simulink model "rtlsdr_fm_fdm_demod"  (R2014b)
settings: Solver=ode45  StartTime=0.0  StopTime=60  RelTol=1e-3
PreLoadFcn:
  | %%%%%%%%%%%%%%%%%%%%%%%%%%%%%%%%%%%%%%%%%%%%%%%%%%%%%%%%%%%%%%%%%%%%%%%%%%%
  | % check to see if Simulink library folder is missing from the MATLAB path %
  | %%%%%%%%%%%%%%%%%%%%%%%%%%%%%%%%%%%%%%%%%%%%%%%%%%%%%%%%%%%%%%%%%%%%%%%%%%%
  | if isempty(strfind(path, 'rtlsdr_book_library'))
  | 
  |     % create error window
  |     fig_error = figure(...
  |         'Name', 'Error: RTL-SDR Book Library',...
  |         'Toolbar','none',...
  |         'MenuBar','none',...
  |         'NumberTitle','off',...
  |         'Resize','off',...
  |         'WindowStyle','modal');
  |     fig_error.Position(3) = 600;
  |     fig_error.Position(4) = 150;
  |     fig_axes = axes(...
  |         'Parent',fig_error,...
  |         'Position',[0,0,1,1],...
  |         'visible','off');
  |     % error message
  |     t_title = text(.05,.8,...
  |         'MISSING DIRECTORIES',...
  |         'FontSize',11.5);
  |     t_body = text(.075,.6,...
  |         [{'Simulink cannot find the  \it{<root>}\rm / \it{rtlsdr\_book\_library}\rm  folder in the \it{MATLAB Path}\rm.'},...
  |         {'Please set the MATLAB path following the instructions given in Exercise 2.4.'}],...
  |         'FontSize',10.5);
  |     % buttons
  |     btn_path = uicontrol(...
  |         'Parent',fig_error,...
  |         'String','Set Path Now',...
  |         'FontSize',10,...
  |         'Callback', 'pathtool; close(fig_error);',...
  |         'Position', [fig_error.Position(3)/2-210, 30, 200, 30]);
  |     btn_abort = uicontrol(...
  |         'Parent',fig_error,...
  |         'String','No thanks',...
  |         'FontSize',10,...
  |         'Callback', 'close(fig_error); abort=1;',...
  |         'Position', [fig_error.Position(3)/2+10, 30, 200, 30]);
  | 
  |     % pause to allow user to interact with error box
  |     uiwait(fig_error);
  | 
  |     % abort simulation
  |     try
  |         if abort==1
  |             set_param(gcs, 'SimulationCommand', 'stop');
  |         end
  |     end
  | 
  |     % if user has set path, allow diagram to be updated
  |     if ~exist('abort','var')
  |         % create error window
  |         fig_update = figure(...
  |             'Name', 'Update Diagram',...
  |             'Toolbar','none',...
  |             'MenuBar','none',...
  |             'NumberTitle','off',...
  |             'Resize','off');
  |         fig_update.Position(3) = 400;
  |         fig_update.Position(4) = 120;
  |         fig_axes = axes(...
  |             'Parent',fig_update,...
  |             'Position',[0,0,1,1],...
  |             'visible','off');
  |         % instruction message
  |         t_body = text(.075,.7,...
  |             'Once you have set the path, update the block diagram',...
  |             'FontSize',10.5);
  |         % button
  |         btn_update = uicontrol(...
  |             'Parent',fig_update,...
  |             'String','Update Block Diagram',...
  |             'FontSize',10,...
  |             'Callback', 'set_param(gcs,''SimulationCommand'',''update''); close(gcf)',...
  |             'Position', [fig_update.Position(3)/2-100, 30, 200, 30]);
  |     end
  | 
  |     % clear error components
  |     clear('fig_error','fig_update','fig_axes','t_title','t_body','btn_path','btn_abort','btn_update','abort');
  | 
  | end
  | %%%%%%%%%%%%%%%%%%%%%%%%%%%%%%%%%%%%%%%%%%%%%%%%%%%%%%%%%%%%%%%%%%%%%%%%%%%
undefined symbols (not defined in the file or in its folder): dfilt, fdesignblkfcn, gcbh, startfcn_spectrum_analyzer
libraries: dsparch4 x5, rtlsdr_book_library x4, dspmlti4 x3, sdrrlib x1, dspsnks4 x1
CloseFcn:
  | closefcn_model
Description:
  | Software, Simulation Examples and Design Exercises Licence Agreement
  | 
  | This license agreement refers to the simulation examples, design exercises and files,
  | and associated software MATLAB and Simulink resources that accompany the book:
  | 
  |      Title: Software Defined Radio using MATLAB & Simulink and the RTL-SDR
  |      Published by Strathclyde Academic Media, 2015
  |      Authored by Robert W. Stewart, Kenneth W. Barlee, Dale S.W. Atkinson,
  |      and Louise H. Crockett
  | 
  | and made available as a download from, www.desktopSDR.com or variously acquired
  | by other means such as via USB storage, cloud storage, disk or any other electronic
  | or optical or magnetic storage mechanism. These files and associated software may
  | be used subject to the terms of agreement of the conditions below:
  | 
  |     Copyright © 2015 Robert W. Stewart, Kenneth W. Barlee, Dale S.W. Atkinson,
  |     and Louise H. Crockett
  |     All rights reserved.
  | 
  | Redistribution and use in source and binary forms, with or without modification, are
  | permitted provided that the following conditions are met:
  | 
  |    1.  Redistributions of source code must retain the above copyright notice, this list of
  |         conditions and the following disclaimer.
  | 
  |    2.  Redistributions in binary form must reproduce the above copyright notice, this
  |         list of conditions and the following disclaimer in the documentation and/or other
  |         materials provided with the distribution.
  | 
  |    3.  Neither the name of the copyright holder nor the names of its contributors may
  |         be used to endorse or promote products derived from this software without
  |         specific prior written permission.
  | 
  |    4.  In all cases, the software is, and all modifications and derivatives of the
  |         software shall be, licensed to you solely for use in conjunction with The
  |         MathWorks, Inc. products and service offerings.
  | 
  | THIS SOFTWARE IS PROVIDED BY THE COPYRIGHT HOLDERS AND CONTRIBUTORS
  | "AS IS" AND ANY EXPRESS OR IMPLIED WARRANTIES, INCLUDING, BUT NOT LIMITED
  | TO, THE IMPLIED WARRANTIES OF MERCHANTABILITY AND FITNESS FOR A
  | PARTICULAR PURPOSE ARE DISCLAIMED. IN NO EVENT SHALL THE COPYRIGHT
  | HOLDER OR CONTRIBUTORS BE LIABLE FOR ANY DIRECT, INDIRECT, INCIDENTAL,
  | SPECIAL, EXEMPLARY, OR CONSEQUENTIAL DAMAGES (INCLUDING, BUT NOT
  | LIMITED TO, PROCUREMENT OF SUBSTITUTE GOODS OR SERVICES; LOSS OF USE,
  | DATA, OR PROFITS; OR BUSINESS INTERRUPTION) HOWEVER CAUSED AND ON ANY
  | THEORY OF LIABILITY, WHETHER IN CONTRACT, STRICT LIABILITY, OR TORT
  | (INCLUDING NEGLIGENCE OR OTHERWISE) ARISING IN ANY WAY OUT OF THE USE
  | OF THIS SOFTWARE, EVEN IF ADVISED OF THE POSSIBILITY OF SUCH DAMAGE.
  | 
  | 
  | Audio Tracks used in Simulations Examples and Design Exercises
  | 
  | The music and vocal files used within the Examples files and software within the book
  | were variously written, arranged, performed, recorded and produced by Garrey Rice,
  | Adam Struth, Jamie Struth, Iain Thistlethwaite and also Marshall Craigmyle who
  | collectively, and individually where appropriate, assert and retain all of their copyright,
  | performance and artistic rights. Permission to use and reproduce this music is
  | granted for all purposes associated with MATLAB and Simulink software and the
  | simulation examples and design exercises files that accompany this book. Requests to
  | use the music for any other purpose should be directed to: info@desktopSDR.com.
  | For information on music track names, full credits, and links to the musicians please
  | refer to www.desktopSDR.com/more/audio.
settings Model: SimulationMode=accelerator  Creator=desktopSDR Team  LastModifiedBy=desktopSDR Team
settings DataIOCC: LimitDataPoints=off  SaveOutput=off  SignalLogging=off  SaveTime=off

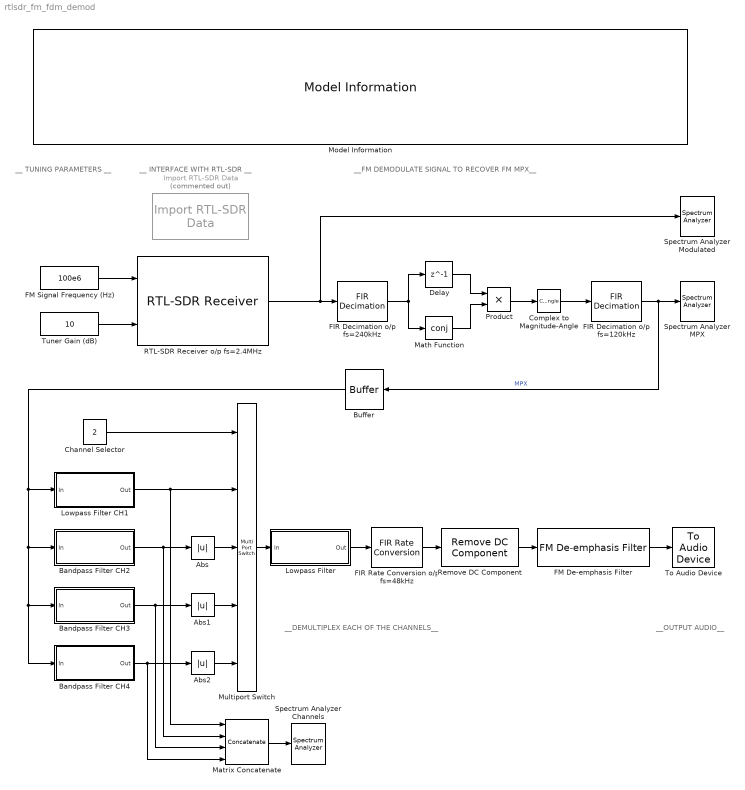
== system rtlsdr_fm_fdm_demod ==
  note: __ TUNING PARAMETERS __
  note: __ INTERFACE WITH RTL-SDR __
  note: __OUTPUT AUDIO__
  note: __FM DEMODULATE SIGNAL TO RECOVER FM MPX__
  note: __DEMULTIPLEX EACH OF THE CHANNELS__
  Abs : Abs
  Abs1 : Abs
  Abs2 : Abs
  Bandpass Filter CH2 : Subsystem  DialogController=fdesignblkfcn  InitFcn=fdesignblkfcn(gcbh, {'InitFcn'});  mask(Bandpass Filter){}
      mask help: Design a bandpass filter
      settings: CopyFcn=fdesignblkfcn(gcbh, {'CopyFcn'});
      mask Help: helpview(mapfilelocation('dsp'), 'dspbandpassfilter');
      mask Display: disp('Bandpass');
  Bandpass Filter CH3 : Subsystem  DialogController=fdesignblkfcn  InitFcn=fdesignblkfcn(gcbh, {'InitFcn'});  mask(Bandpass Filter){}
      mask help: Design a bandpass filter
      settings: CopyFcn=fdesignblkfcn(gcbh, {'CopyFcn'});
      mask Help: helpview(mapfilelocation('dsp'), 'dspbandpassfilter');
      mask Display: disp('Bandpass');
  Bandpass Filter CH4 : Subsystem  DialogController=fdesignblkfcn  InitFcn=fdesignblkfcn(gcbh, {'InitFcn'});  mask(Bandpass Filter){}
      mask help: Design a bandpass filter
      settings: CopyFcn=fdesignblkfcn(gcbh, {'CopyFcn'});
      mask Help: helpview(mapfilelocation('dsp'), 'dspbandpassfilter');
      mask Display: disp('Bandpass');
  Buffer : Buffer  N=4000  TreatMby1Signals=One channel
  Channel Selector : Constant  Value=2
  Complex to Magnitude-Angle : ComplexToMagnitudeAngle  Output=Angle
  Delay : Delay  DelayLength=1  InitialCondition=0  InputProcessing=Columns as channels (frame based)
  FIR Decimation o/p fs=120kHz : dspmlti4/FIR Decimation  h=firpm(150, [0 53e3 60e3 (240e3/2)]/(240e3/2), [1 1 0 0], [1 1],20)  D=2  filtStruct=Direct form  framing=Allow multirate processing  inputOffset=0  outputBufInitCond=0  InputProcessing=Columns as channels (frame based)  firstCoeffDataTypeStr=Inherit: Same word length as input  firstCoeffLastDataTypeStr=Inherit: Same word length as input  firstCoeffMin=[]  firstCoeffMax=[]  outputDataTypeStr=Inherit: Same as accumulator  outputLastDataTypeStr=Inherit: Same as accumulator  outputMin=[]  outputMax=[]  roundingMode=Floor  overflowMode=off  FilterSource=Specify via dialog  FilterObject=Hm_firdecim
      settings: allowOverrides=off
  FIR Decimation o/p fs=240kHz : dspmlti4/FIR Decimation  h=firpm(50, [0 120e3 240e3 (2.4e6/2)]/(2.4e6/2), [1 1 0 0], [1 1],20)  D=10  filtStruct=Direct form  framing=Allow multirate processing  inputOffset=0  outputBufInitCond=0  InputProcessing=Columns as channels (frame based)  firstCoeffDataTypeStr=Inherit: Same word length as input  firstCoeffLastDataTypeStr=Inherit: Same word length as input  firstCoeffMin=[]  firstCoeffMax=[]  outputDataTypeStr=Inherit: Same as accumulator  outputLastDataTypeStr=Inherit: Same as accumulator  outputMin=[]  outputMax=[]  roundingMode=Floor  overflowMode=off  FilterSource=Specify via dialog  FilterObject=Hm_firdecim
      settings: allowOverrides=off
  FIR Rate Conversion o/p fs=48kHz : dspmlti4/FIR Rate Conversion  L=2  h=firpm(150, [0 5e3 10e3 240e3/2]/(240e3/2), [1 1 0 0], [1 1],20)  M=5  firstCoeffDataTypeStr=Inherit: Same word length as input  firstCoeffLastDataTypeStr=Inherit: Same word length as input  firstCoeffMin=[]  firstCoeffMax=[]  outputDataTypeStr=Inherit: Same as accumulator  outputLastDataTypeStr=Inherit: Same as accumulator  outputMin=[]  outputMax=[]  roundingMode=Floor  overflowMode=off  FilterSource=Specify via dialog  FilterObject=Hm_firsrc
  FM De-emphasis Filter : rtlsdr_book_library/FM Demod Tools/FM De-emphasis Filter  region=Europe, Asia  fs=48e3
  FM Signal Frequency (Hz) : Constant  Value=100e6
  Import RTL-SDR Data : rtlsdr_book_library/Additional Tools/Import RTL-SDR Data  Commented=on  filename=rec_data/wfm_fmfdm.mat  frm_size=4096  data_type=single
  Lowpass Filter : Subsystem  DialogController=fdesignblkfcn  InitFcn=fdesignblkfcn(gcbh, {'InitFcn'});  mask(Lowpass Filter){}
      mask help: Design a lowpass filter
      settings: CopyFcn=fdesignblkfcn(gcbh, {'CopyFcn'});
      mask Help: helpview(mapfilelocation('dsp'), 'dsplowpassfilter');
      mask Display: disp('Lowpass')
  Lowpass Filter CH1 : Subsystem  DialogController=fdesignblkfcn  InitFcn=fdesignblkfcn(gcbh, {'InitFcn'});  mask(Lowpass Filter){}
      mask help: Design a lowpass filter
      settings: CopyFcn=fdesignblkfcn(gcbh, {'CopyFcn'});
      mask Help: helpview(mapfilelocation('dsp'), 'dsplowpassfilter');
      mask Display: disp('Lowpass')
  Math Function : Math  Operator=conj  SaturateOnIntegerOverflow=on
  Matrix Concatenate : Concatenate  NumInputs=4  Mode=Multidimensional array  ConcatenateDimension=2
  Model Information : rtlsdr_book_library/Additional Tools/Model Information/Model Information
  Multiport Switch : MultiPortSwitch  Inputs=4
  Product : Product
  RTL-SDR Receiver o/p fs=2.4MHz : sdrrlib/RTL-SDR Receiver  SourceLibraryInfo="This block requires <a href=\"http://www.mathworks.com/hardware-support/rtl-sdr.html\">Communications System Toolbox Support Package for RTL-SDR Radio</a>"  sobjType=sdrr.internal.SDRRTLReceiverSL  IPAddress=0  dataUDPPort=-1  ctrlUDPPort=-1  subDeviceList=nosubdev  sdrBlockType=SDRBlockTypeSLT.SDRRxBlock  requester=UNUSED_BY_SFCN  sdrExecutionMode=SDRExecutionModeSLT.ExecModeHW  LostSamplesOutputPort=off  OutputDataType=single  FrameLength=4096  EnableBurstMode=off  NumFramesInBurst=20  BypassUserLogic=off  DecimatorSelect=DDC decimator  SourceSelect=RF data  SineAmplitude=16000  EnableInternalClock=off  BypassIQBalance=off  CenterFrequency=100e6  IFBandwidth=40e6  ADCRateSource=Dialog  ADCRate=2.4e6  CenterFrequencySource=Input port  GainSource=Input port  IntermediateFrequency=0  Gain=25  DecimationFactorSource=Dialog  DecimationFactor=512  RFFrequencyIsTunable=logical(1)  SampleTime=(4096)/(2.4e6)  IFBandwidthSource=Dialog  SineFrequency=30000  BypassDCBlockingFilter=off  IntermediateFrequencySource=Dialog  IQBalanceCoefficients=64  SkipAllHardwareResetAndInitialization=off  EnableIQCalibrationTable=on  CacheIQCalibrationTable=off  EnableOffsetTuning=off  EnableRTLAGC=off  EnableTestMode=off  EnableTunerAGC=off  FrequencyCorrectionSource=Dialog  FrequencyCorrection=0  NumMLBuffers=128  NumUSBBuffers=16  LatencyOutputPort=off  RTLCrystalFrequency=28800000  TunerCrystalFrequency=28800000
  Remove DC Component : rtlsdr_book_library/Additional Tools/Remove DC Component
  Spectrum Analyzer Channels : SpectrumAnalyzer  StartFcn=startfcn_spectrum_analyzer;
  Spectrum Analyzer MPX : SpectrumAnalyzer  StartFcn=startfcn_spectrum_analyzer;
  Spectrum Analyzer Modulated : SpectrumAnalyzer  StartFcn=startfcn_spectrum_analyzer;
  To Audio Device : dspsnks4/To Audio Device  deviceName=Default  inheritSampleRate=on  sampleRate=44100  deviceDatatype=Determine from input data type  autoBufferSize=on  bufferSize=4096  queueDuration=1.0  defaultOutputChannelMapping=on  outputChannelMapping=1  outputNumUnderrunSamples=off
  Tuner Gain (dB) : Constant  Value=10
  wires:
  Delay/1 -> Product/1
  Math Function/1 -> Product/2
  Product/1 -> Complex to Magnitude-Angle/1
  FIR Decimation o/p fs=120kHz/1 -> Buffer/1, Spectrum Analyzer MPX/1  "MPX"
  Tuner Gain (dB)/1 -> RTL-SDR Receiver o/p fs=2.4MHz/2
  FM Signal Frequency (Hz)/1 -> RTL-SDR Receiver o/p fs=2.4MHz/1
  RTL-SDR Receiver o/p fs=2.4MHz/1 -> Spectrum Analyzer Modulated/1, FIR Decimation o/p fs=240kHz/1
  FIR Decimation o/p fs=240kHz/1 -> Delay/1, Math Function/1
  Complex to Magnitude-Angle/1 -> FIR Decimation o/p fs=120kHz/1
  Bandpass Filter CH2/1(Out) -> Matrix Concatenate/2, Abs/1
  Lowpass Filter CH1/1(Out) -> Multiport Switch/2, Matrix Concatenate/1
  Channel Selector/1 -> Multiport Switch/1
  Bandpass Filter CH4/1(Out) -> Abs2/1, Matrix Concatenate/4
  Matrix Concatenate/1 -> Spectrum Analyzer Channels/1
  Abs/1 -> Multiport Switch/3
  Bandpass Filter CH3/1(Out) -> Abs1/1, Matrix Concatenate/3
  Abs2/1 -> Multiport Switch/5
  Multiport Switch/1 -> Lowpass Filter/1(In)
  Buffer/1 -> Bandpass Filter CH3/1(In), Bandpass Filter CH4/1(In), Bandpass Filter CH2/1(In), Lowpass Filter CH1/1(In)
  Abs1/1 -> Multiport Switch/4
  FM De-emphasis Filter/1 -> To Audio Device/1
  Lowpass Filter/1(Out) -> FIR Rate Conversion o/p fs=48kHz/1
  Remove DC Component/1 -> FM De-emphasis Filter/1
  FIR Rate Conversion o/p fs=48kHz/1 -> Remove DC Component/1

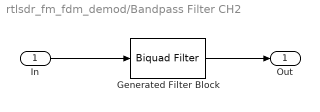
== system rtlsdr_fm_fdm_demod/Bandpass Filter CH2 ==
  In : Inport
  Generated Filter Block : dsparch4/Biquad Filter  Tag=BlockMethodSubSystem  IIRFiltStruct=Direct form II  CoeffSource=Specify via dialog  BiQuadCoeffs=[0.14648306875469183 -0.013426158327361541 0.12850352494747963 1 -1.4524452044662892 0.93045107330293608;0.040274452848524468 0.00070941875773438323 0.029497628365742094 1 -1.7980790998083904 0.90832465933463091;0.12049657869797133 0.0044347373173777354 8.5134870626890966e-06 1 -1.7109902214647215 0.87168820603812525;0.22074995540315487 0.17447437418812073 0.02596198322321908 1 -1.6271379063210059 0.86160411775111889;-0.019372943183859893 0.0273115235436748 -0.019372832365970961 1 -1.4387264332701792 0.98945943815018489;1.0345735931099562 -2 1.0345529044927504 1 -1.9084943451375511 0.98834226659913782;1.9999999999999998 0.73469996927398884 0.43067824988310621 1 -1.491948381136623 0.89803675911009373;0.51905980407287411 -0.10905354623743906 0.0046837415732670076 1 -1.5523022673081051 0.87294845610455429;0.86595616600144976 -1.6879989072243624 0.86661849715818873 1 -1.4364798170683248 0.96333880696279617;1.1930528438977974 -0.20649886676264312 0.010039403489850742 1 -1.869133466821796 0.9557124313304397]  a0Flag=Warning  IC=0  ICnum=0  ICden=0  InputProcessing=Columns as channels (frame based)  denAccumFracLength=30  denProdOutputFracLength=30  secondMemoryFracLength=15  roundingMode=Floor  overflowMode=off  ScaleValues=[0.045774778457568492;1;1;1;1;1;1;1;1;1;1]  optimizeScaleValues=off  ScaleValueMode=Specify via input port (g)  scaleValueFracLength=14  FilterSource=Specify via dialog  dfiltObjectName=dfilt.df2tsos([1 0.3 0.4],[1 0.1 0.2])
  Out : Outport
  wires:
  Generated Filter Block/1 -> Out/1
  In/1 -> Generated Filter Block/1

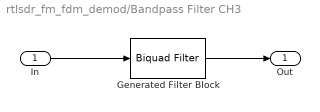
== system rtlsdr_fm_fdm_demod/Bandpass Filter CH3 ==
  In : Inport
  Generated Filter Block : dsparch4/Biquad Filter  Tag=BlockMethodSubSystem  IIRFiltStruct=Direct form II  CoeffSource=Specify via dialog  BiQuadCoeffs=[0.47686243400571915 -0.10116708683355603 0.46498608051198081 1 0.40578328206191572 0.92121270016476908;0.72162735121003008 0.97957713509778521 0.70763391787358054 1 1.1187126037088988 0.91408420208689445;0.37789284276504836 0.3178346722839 0.066814940759488808 1 0.63117562805836425 0.82009857191240298;0.019927573205180227 -0.011105358924836429 0.00027793213458167018 1 0.81024145786390034 0.80942592856636275;2 0.61866154498158576 1.9996942814570717 1 0.35423720417521776 0.99004875427963779;1.5861746157751597 2 1.5851537007699816 1 1.2184838877095743 0.98987622169272638;0.74034429252258405 -0.2875225404483055 0.50463041164383216 1 0.49120076094257603 0.86649366035041653;0.032094327865033266 -0.045623467796807704 0.02478046341084213 1 0.98828882445532196 0.84944830200910626;0.68806539584499549 0.18672509929123804 0.68673147904723819 1 0.36645001611784678 0.96372056765640113;1.5578400672155699 2 1.5465281770553045 1 1.1881132879801917 0.96235975455813594]  a0Flag=Warning  IC=0  ICnum=0  ICden=0  InputProcessing=Columns as channels (frame based)  denAccumFracLength=30  denProdOutputFracLength=30  secondMemoryFracLength=15  roundingMode=Floor  overflowMode=off  ScaleValues=[0.07700689545937929;1;1;1;1;1;1;1;1;1;9.1631392145887141]  optimizeScaleValues=off  ScaleValueMode=Specify via input port (g)  scaleValueFracLength=14  FilterSource=Specify via dialog  dfiltObjectName=dfilt.df2tsos([1 0.3 0.4],[1 0.1 0.2])
  Out : Outport
  wires:
  In/1 -> Generated Filter Block/1
  Generated Filter Block/1 -> Out/1

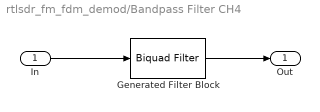
== system rtlsdr_fm_fdm_demod/Bandpass Filter CH4 ==
  In : Inport
  Generated Filter Block : dsparch4/Biquad Filter  Tag=BlockMethodSubSystem  IIRFiltStruct=Direct form II  CoeffSource=Specify via dialog  BiQuadCoeffs=[1.0077722767661659 2 0.99228766163190596 1 1.73684022311522 0.91986702489055161;0.63792313072434204 1.2712205257033025 0.63330258372394233 1 1.3070120975180517 0.89326942633878648;1.2946681784251903 0.079101636184802412 0.0010965548460564892 1 1.5125481836192141 0.84185080733317819;0.029036155911700303 -0.012007507809340947 0.00035949003154971945 1 -0.31125861506850827 0.012931195809741119;0.42656461871431595 0.79741819277571147 0.42655905180147818 1 1.8399523823767157 0.98893127818608106;1.5941851626132932 2 1.5941720895408855 1 1.2852927977662061 0.98780160835756381;-1.531097744961885 -1.878832896803069 -0.3285338306777269 1 1.6379806104358501 0.87494578709400117;0.093767433948846415 0.013621498750544948 0.00045772176218882423 1 1.3879691565418619 0.84511312428391383;0.81139017858721285 0.97789780072477561 0.81051462769961502 1 1.8028771594647566 0.96017308577394067;1.0796313891798923 2 0.92210137226894129 1 1.2828686017719715 0.95180413582849388]  a0Flag=Warning  IC=0  ICnum=0  ICden=0  InputProcessing=Columns as channels (frame based)  denAccumFracLength=30  denProdOutputFracLength=30  secondMemoryFracLength=15  roundingMode=Floor  overflowMode=off  ScaleValues=[0.034011689091950244;1;1;1;1;1;1;1;1;1;6.1582128506267733]  optimizeScaleValues=off  ScaleValueMode=Specify via input port (g)  scaleValueFracLength=14  FilterSource=Specify via dialog  dfiltObjectName=dfilt.df2tsos([1 0.3 0.4],[1 0.1 0.2])
  Out : Outport
  wires:
  In/1 -> Generated Filter Block/1
  Generated Filter Block/1 -> Out/1

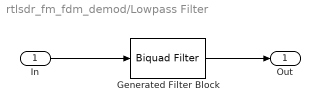
== system rtlsdr_fm_fdm_demod/Lowpass Filter ==
  In : Inport
  Generated Filter Block : dsparch4/Biquad Filter  Tag=BlockMethodSubSystem  IIRFiltStruct=Direct form II  CoeffSource=Specify via dialog  BiQuadCoeffs=[1.1405548261092002 -2 0.99774384818807205 1 -1.6151678875945503 0.61545058918626938;2 0.11048867543151997 -0.009553237706361602 1 -0.39423132078966727 0.038591162384855944;0.4007465992983309 0.50117026640197415 0.15242239003559271 1 -0.041388616066048378 -0.010386157974634323;0.087152346143881579 -0.07866330613938588 0.044403621140389302 1 -0.58363069553949543 0.085015456031925854;1.0437992027798593 -2 1.0358419331721138 1 -1.9133920037763108 0.96628466492119591;1.8222894236479241 0.76771223538764566 2 1 0.015097687434627471 -0.35980889568685881;0.79320057311859937 0.34483454382067436 0.027321918127832658 1 -0.26856139709736748 0.018031302075906329;2 -0.23965551507121227 -1.7591017238423925 1 -0.13717476892986813 0.0045806304277620138;1.6684992485747192 -2 1.2868514556028745 1 -0.4882437965019687 0.059483334188892276;2 1.4576569898159009 1.4370562165856733 1 0.79243004979363274 0.91392237461091153]  a0Flag=Warning  IC=0  ICnum=0  ICden=0  InputProcessing=Columns as channels (frame based)  denAccumFracLength=30  denProdOutputFracLength=30  secondMemoryFracLength=15  roundingMode=Floor  overflowMode=off  ScaleValues=[0.00028270159171905895;1;1;1;1;1;1;1;1;1;133.01324553146722]  optimizeScaleValues=off  ScaleValueMode=Specify via input port (g)  scaleValueFracLength=14  FilterSource=Specify via dialog  dfiltObjectName=dfilt.df2tsos([1 0.3 0.4],[1 0.1 0.2])
  Out : Outport
  wires:
  In/1 -> Generated Filter Block/1
  Generated Filter Block/1 -> Out/1

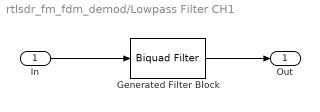
== system rtlsdr_fm_fdm_demod/Lowpass Filter CH1 ==
  In : Inport
  Generated Filter Block : dsparch4/Biquad Filter  Tag=BlockMethodSubSystem  IIRFiltStruct=Direct form II  CoeffSource=Specify via dialog  BiQuadCoeffs=[1.1405548261092002 -2 0.99774384818807205 1 -1.6151678875945503 0.61545058918626938;2 0.11048867543151997 -0.009553237706361602 1 -0.39423132078966727 0.038591162384855944;0.4007465992983309 0.50117026640197415 0.15242239003559271 1 -0.041388616066048378 -0.010386157974634323;0.087152346143881579 -0.07866330613938588 0.044403621140389302 1 -0.58363069553949543 0.085015456031925854;1.0437992027798593 -2 1.0358419331721138 1 -1.9133920037763108 0.96628466492119591;1.8222894236479241 0.76771223538764566 2 1 0.015097687434627471 -0.35980889568685881;0.79320057311859937 0.34483454382067436 0.027321918127832658 1 -0.26856139709736748 0.018031302075906329;2 -0.23965551507121227 -1.7591017238423925 1 -0.13717476892986813 0.0045806304277620138;1.6684992485747192 -2 1.2868514556028745 1 -0.4882437965019687 0.059483334188892276;2 1.4576569898159009 1.4370562165856733 1 0.79243004979363274 0.91392237461091153]  a0Flag=Warning  IC=0  ICnum=0  ICden=0  InputProcessing=Columns as channels (frame based)  denAccumFracLength=30  denProdOutputFracLength=30  secondMemoryFracLength=15  roundingMode=Floor  overflowMode=off  ScaleValues=[0.00028270159171905895;1;1;1;1;1;1;1;1;1;133.01324553146722]  optimizeScaleValues=off  ScaleValueMode=Specify via input port (g)  scaleValueFracLength=14  FilterSource=Specify via dialog  dfiltObjectName=dfilt.df2tsos([1 0.3 0.4],[1 0.1 0.2])
  Out : Outport
  wires:
  Generated Filter Block/1 -> Out/1
  In/1 -> Generated Filter Block/1
